simulink library "autodiff"  (R2017a)
settings: Solver=ode45  StartTime=0.0  StopTime=10.0  RelTol=1e-3  EnableMultiTasking=on
undefined symbols (not defined in the file or in its folder): trace
libraries: autodiff x19
settings Model: Creator=eruffaldi  LastModifiedBy=eruffaldi
settings DataIOCC: LimitDataPoints=on
settings OptimizationCC: LifeSpan=inf
settings DebuggingCC: AllowSymbolicDim=off  SFUnexpectedBacktrackingDiag=warning  SFNoUnconditionalDefaultTransitionDiag=warning  SFExecutionAtInitializationDiag=none
settings GRTTargetCC: TargetLangStandard=C89/C90 (ANSI)  GeneratePreprocessorConditionals=Disable all
settings ConfigComp: CovMetricSettings=dw  CovHtmlReporting=on  CovSaveCumulativeToWorkspaceVar=on  CovSaveSingleToWorkspaceVar=on  CovExternalEMLEnable=off

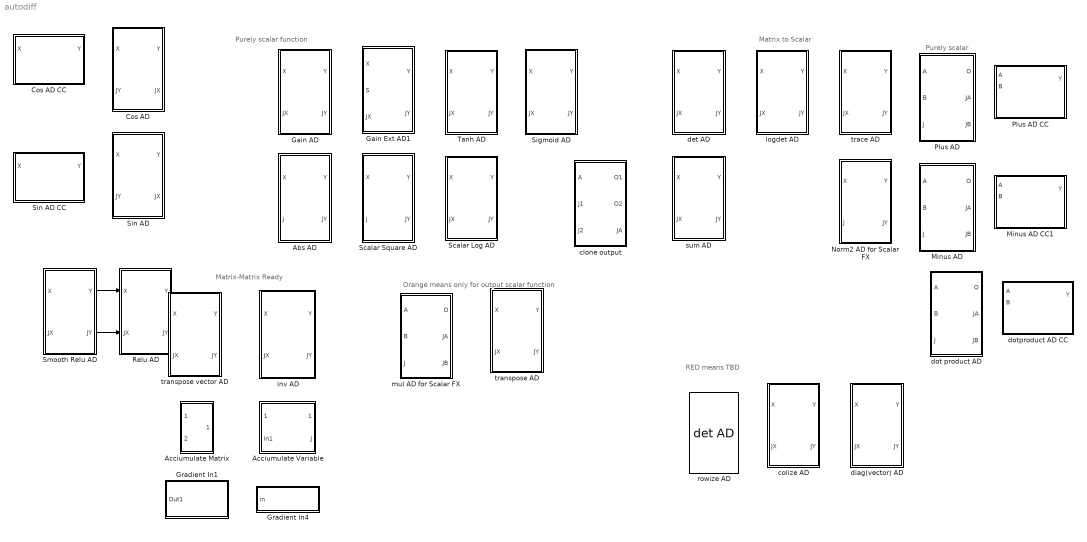
== system autodiff ==
  note: Matrix-Matrix Ready
  note: Purely scalar
  note: Matrix to Scalar
  note: Purely scalar function
  note: Orange means only for output scalar function
  note: RED means TBD
  Abs AD : Subsystem
  Acciumulate Matrix : Subsystem  mask{Inputs=2}
      mask Callback Inputs:
      | x = gcb;
      | s = gcb;
      | asked = max(1,str2num(get_param(gcb,'Inputs')));
      | 
      | bcon = [x '/Matrix Concatenate'];
      | actual = str2num(get_param(bcon,'NumInputs'));
      | 
      | if asked == actual
      | else
      | bconL = bcon(length(x)+2:end);
      | 
      | if asked > actual
      |     set_param(bcon,'NumInputs',num2str(asked));
      |     bin1 = ([x '/In1']);
      |     bsh1 = ([x '/Reshape1']);
      |     bin1L = bin1(length(x)+2:end);
      |     bsh1L = bsh1(length(x)+2:end);
      |     for I=actual+1:asked
      |         bin = sprintf([x '/In%d'],I);
      |         bsh = sprintf([x '/Reshape%d'],I);
      |         binL = bin(length(x)+2:end);
      |         bshL = bsh(length(x)+2:end);
      |         % clone In and Reshape
      |         add_block(bin1,bin);
      |         add_block(bsh1,bsh);
      |         add_line(s,[binL '/1'],[bshL '/1']);
      |         add_line(s,[bshL '/1'],[bconL sprintf('/%d',I)]);
      |     end
      | else
      |     % remove
      |     for I=actual:-1:asked+1
      |         bin = sprintf([x '/In%d'],I);
      |         bsh = sprintf([x '/Reshape%d'],I);
      |         binL = bin(length(x)+2:end);
      |         bshL = bsh(length(x)+2:end);
      | 
      |         try
      |         delete_line(s,[binL '/1'],[bshL '/1']);
      |         catch me
      |         end
      |         try
      |         delete_line(s,[bshL '/1'],[bconL sprintf('/%d',I)]);
      |         catch me
      |         end
      |         try
      |         delete_block(bin);
      |         catch me
      |         end
      |         try
      |         delete_block(bsh);
      |         catch me
      |         end
      |     end
      |     set_param(bcon,'NumInputs',num2str(asked));
      | end
      | end
  Acciumulate Variable : Subsystem  mask{Inputs=1}
      mask Callback Inputs:
      | x = gcb;
      | s = gcb;
      | asked = max(1,str2num(get_param(gcb,'Inputs')));
      | 
      | bcon = [x '/Matrix Concatenate'];
      | actual = str2num(get_param(bcon,'NumInputs'));
      | 
      | if asked == actual
      | else
      | bconL = bcon(length(x)+2:end);
      | 
      | if asked > actual
      |     set_param(bcon,'NumInputs',num2str(asked));
      |     bin1 = ([x '/In1']);
      |     bsh1 = ([x '/Reshape1']);
      |     bin1L = bin1(length(x)+2:end);
      |     bsh1L = bsh1(length(x)+2:end);
      |     for I=actual+1:asked
      |         bin = sprintf([x '/In%d'],I);
      |         bsh = sprintf([x '/Reshape%d'],I);
      |         binL = bin(length(x)+2:end);
      |         bshL = bsh(length(x)+2:end);
      |         % clone In and Reshape
      |         add_block(bin1,bin);
      |         add_block(bsh1,bsh);
      |         add_line(s,[binL '/1'],[bshL '/1']);
      |         add_line(s,[bshL '/1'],[bconL sprintf('/%d',I)]);
      |     end
      | else
      |     % remove
      |     for I=actual:-1:asked+1
      |         bin = sprintf([x '/In%d'],I);
      |         bsh = sprintf([x '/Reshape%d'],I);
      |         binL = bin(length(x)+2:end);
      |         bshL = bsh(length(x)+2:end);
      | 
      |         try
      |         delete_line(s,[binL '/1'],[bshL '/1']);
      |         catch me
      |         end
      |         try
      |         delete_line(s,[bshL '/1'],[bconL sprintf('/%d',I)]);
      |         catch me
      |         end
      |         try
      |         delete_block(bin);
      |         catch me
      |         end
      |         try
      |         delete_block(bsh);
      |         catch me
      |         end
      |     end
      |     set_param(bcon,'NumInputs',num2str(asked));
      | end
      | end
  Cos AD : Subsystem
  Cos AD CC : Subsystem
  Gain AD : Subsystem  mask{k=1}
      mask prompts: k "Gain Constant"
  Gain Ext AD1 : Subsystem
  Gradient In1 : Subsystem
  Gradient In4 : Subsystem
  Minus AD : Subsystem
  Minus AD CC1 : Subsystem
  Norm2 AD for Scalar FX : Subsystem
  "Plus AD " : Subsystem
  Plus AD CC : Subsystem
  Relu AD : Subsystem
  Scalar Log AD : Subsystem
  Scalar Square AD : Subsystem
  Sigmoid AD : Subsystem
  Sin AD : Subsystem
  Sin AD CC : Subsystem
  Smooth Relu AD : Subsystem
  Tanh AD : Subsystem
  clone output : Subsystem
  colize AD : Subsystem
  det AD : Subsystem
  diag(vector) AD : Subsystem
  dot product AD : Subsystem
  dotproduct AD CC : Subsystem
  inv AD : Subsystem
  logdet AD : Subsystem
  mul AD for Scalar FX : Subsystem
  rowize AD : autodiff/det AD
  sum AD : Subsystem
  trace AD : Subsystem
  transpose AD : Subsystem
  transpose vector AD : Subsystem
  wires:
  Smooth Relu AD/1(Y) -> Relu AD/1(X)
  Smooth Relu AD/2(JY) -> Relu AD/2(JX)

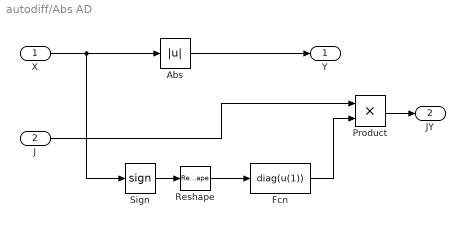
== system autodiff/Abs AD ==
  X : Inport
  J : Inport  Port=2
  Abs : Abs
  Fcn : Fcn  Expr=diag(u(1))
  Product : Product
  Reshape : Reshape  OutputDimensionality=Column vector (2-D)
  Sign : Signum
  Y : Outport
  JY : Outport  Port=2
  wires:
  Abs/1 -> Y/1
  X/1 -> Sign/1, Abs/1
  Sign/1 -> Reshape/1
  Product/1 -> JY/1
  Reshape/1 -> Fcn/1
  J/1 -> Product/1
  Fcn/1 -> Product/2

== system autodiff/Acciumulate Matrix ==
  In1 : Inport
  In2 : Inport  Port=2
  Matrix Concatenate : Concatenate  Mode=Multidimensional array  ConcatenateDimension=2
  Reshape1 : Reshape
  Reshape2 : Reshape
  ReshapeX : Reshape  OutputDimensionality=Derive from reference input port
  Sum of Elements : Sum  Inputs=+  CollapseMode=Specified dimension  CollapseDim=2
  Out1 : Outport
  wires:
  Sum of Elements/1 -> ReshapeX/1
  In1/1 -> ReshapeX/2, Reshape1/1
  Reshape1/1 -> Matrix Concatenate/1
  Matrix Concatenate/1 -> Sum of Elements/1
  ReshapeX/1 -> Out1/1
  In2/1 -> Reshape2/1
  Reshape2/1 -> Matrix Concatenate/2

== system autodiff/Acciumulate Variable ==
  note: InValue is the X that is passed by just due to visual style and it is size [m,n]
      |
      | The In# is automatically populated and it should be [p,q,m,n] that is [pq,mn] we
      | receive a set of k contributions [pq,mn] flatten as [pq mn, 1] then concatenate to [pq mn,k]
      | and sum obtaining as output [pq,mn] again
  InValue : Inport
  In1 : Inport  Port=2
  Matrix Concatenate : Concatenate  NumInputs=1  Mode=Multidimensional array  ConcatenateDimension=2
  Reshape1 : Reshape
  ReshapeX : Reshape  OutputDimensionality=Derive from reference input port
  Sum of Elements : Sum  Inputs=+  CollapseMode=Specified dimension  CollapseDim=2
  OutValue : Outport
  J : Outport  Port=2
  wires:
  Sum of Elements/1 -> ReshapeX/1
  In1/1 -> ReshapeX/2, Reshape1/1
  Reshape1/1 -> Matrix Concatenate/1
  Matrix Concatenate/1 -> Sum of Elements/1
  ReshapeX/1 -> J/1
  InValue/1 -> OutValue/1

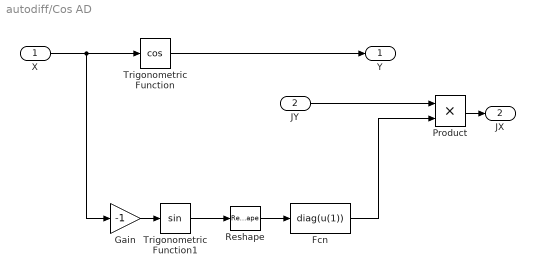
== system autodiff/Cos AD ==
  X : Inport
  JY : Inport  Port=2
  Fcn : Fcn  Expr=diag(u(1))
  Gain : Gain  Gain=-1
  Product : Product
  Reshape : Reshape  OutputDimensionality=Column vector (2-D)
  Trigonometric Function : Trigonometry  Operator=cos
  Trigonometric Function1 : Trigonometry
  Y : Outport
  JX : Outport  Port=2
  wires:
  Trigonometric Function/1 -> Y/1
  X/1 -> Gain/1, Trigonometric Function/1
  Product/1 -> JX/1
  Gain/1 -> Trigonometric Function1/1
  Trigonometric Function1/1 -> Reshape/1
  Fcn/1 -> Product/2
  JY/1 -> Product/1
  Reshape/1 -> Fcn/1

== system autodiff/Cos AD CC ==
  X : Inport
  Cos AD1 : autodiff/Cos AD
  Gradient In2 : autodiff/Gradient In4
  Gradient In3 : autodiff/Gradient In1
  JX : PMIOPort  Port=1  Side=Left
  JY : PMIOPort  Port=2  Side=Right
  Y : Outport
  wires:
  Gradient In3/1 -> Cos AD1/2
  Cos AD1/1 -> Y/1
  X/1 -> Cos AD1/1
  Cos AD1/2 -> Gradient In2/1
  connections:
  Gradient In2/RConn1 -- JX/RConn1
  Gradient In3/LConn1 -- JY/RConn1

== system autodiff/Gain AD ==
  X : Inport
  JX : Inport  Port=2
  Gain1 : Gain  Gain=k
  Gain2 : Gain  Gain=k
  Y : Outport
  JY : Outport  Port=2
  wires:
  Gain1/1 -> Y/1
  X/1 -> Gain1/1
  Gain2/1 -> JY/1
  JX/1 -> Gain2/1

== system autodiff/Gain Ext AD1 ==
  X : Inport
  S : Inport  Port=2
  JX : Inport  Port=3
  Product : Product
  Product1 : Product
  Signal Specification : SignalSpecification  Dimensions=1
  Y : Outport
  JY : Outport  Port=2
  wires:
  Product1/1 -> Y/1
  X/1 -> Product1/1
  Product/1 -> JY/1
  JX/1 -> Product/2
  S/1 -> Signal Specification/1
  Signal Specification/1 -> Product1/2, Product/1

== system autodiff/Gradient In1 ==
  Ground : Ground
  Two-Way Connection : TwoWayConnection
  J out : PMIOPort  Port=1  Side=Left
  Out1 : Outport
  wires:
  Two-Way Connection/1 -> Out1/1
  Ground/1 -> Two-Way Connection/1
  connections:
  J out/RConn1 -- Two-Way Connection/RConn1

== system autodiff/Gradient In4 ==
  " in" : Inport
  Terminator : Terminator
  Two-Way Connection : TwoWayConnection
  J out : PMIOPort  Port=1  Side=Right
  wires:
  " in"/1 -> Two-Way Connection/1
  Two-Way Connection/1 -> Terminator/1
  connections:
  J out/RConn1 -- Two-Way Connection/RConn1

== system autodiff/Minus AD ==
  A : Inport
  B : Inport  Port=2
  J : Inport  Port=3
  Add : Sum  Inputs=+-
  Gain : Gain  Gain=-1
  O : Outport
  JA : Outport  Port=2
  JB : Outport  Port=3
  wires:
  Add/1 -> O/1
  A/1 -> Add/1
  B/1 -> Add/2
  J/1 -> Gain/1, JA/1
  Gain/1 -> JB/1

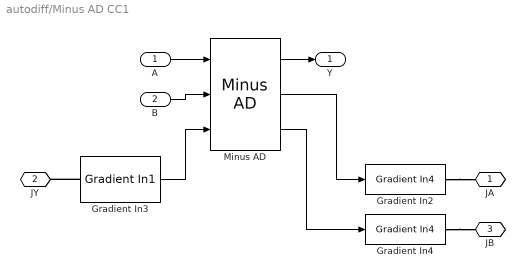
== system autodiff/Minus AD CC1 ==
  A : Inport
  B : Inport  Port=2
  Gradient In2 : autodiff/Gradient In4
  Gradient In3 : autodiff/Gradient In1
  Gradient In4 : autodiff/Gradient In4
  Minus AD : autodiff/Minus AD
  JA : PMIOPort  Port=1  Side=Left
  JY : PMIOPort  Port=2  Side=Right
  JB : PMIOPort  Port=3  Side=Left
  Y : Outport
  wires:
  Gradient In3/1 -> Minus AD/3
  Minus AD/1 -> Y/1
  A/1 -> Minus AD/1
  B/1 -> Minus AD/2
  Minus AD/2 -> Gradient In2/1
  Minus AD/3 -> Gradient In4/1
  connections:
  Gradient In2/RConn1 -- JA/RConn1
  Gradient In3/LConn1 -- JY/RConn1
  Gradient In4/RConn1 -- JB/RConn1

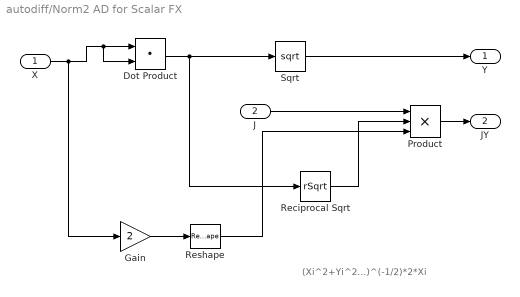
== system autodiff/Norm2 AD for Scalar FX ==
  note: (Xi^2+Yi^2...)^(-1/2)*2*Xi
  X : Inport
  J : Inport  Port=2
  Dot Product : DotProduct  InputSameDT=on  OutDataTypeStr=Inherit: Inherit via internal rule
  Gain : Gain  Gain=2
  Product : Product  Inputs=3
  Reciprocal Sqrt : Sqrt  Operator=rSqrt  SaturateOnIntegerOverflow=on
  Reshape : Reshape  OutputDimensionality=Row vector (2-D)
  Sqrt : Sqrt  SaturateOnIntegerOverflow=on
  Y : Outport
  JY : Outport  Port=2
  wires:
  X/1 -> Gain/1, Dot Product/2, Dot Product/1
  Product/1 -> JY/1
  Dot Product/1 -> Reciprocal Sqrt/1, Sqrt/1
  Sqrt/1 -> Y/1
  J/1 -> Product/1
  Reciprocal Sqrt/1 -> Product/2
  Gain/1 -> Reshape/1
  Reshape/1 -> Product/3

== system autodiff/Plus AD  ==
  A : Inport
  B : Inport  Port=2
  J : Inport  Port=3
  Add : Sum
  O : Outport
  JA : Outport  Port=2
  JB : Outport  Port=3
  wires:
  Add/1 -> O/1
  A/1 -> Add/1
  B/1 -> Add/2
  J/1 -> JB/1, JA/1

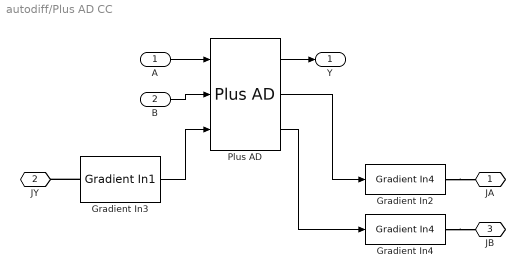
== system autodiff/Plus AD CC ==
  A : Inport
  B : Inport  Port=2
  Gradient In2 : autodiff/Gradient In4
  Gradient In3 : autodiff/Gradient In1
  Gradient In4 : autodiff/Gradient In4
  "Plus AD " : autodiff/Plus AD  
  JA : PMIOPort  Port=1  Side=Left
  JY : PMIOPort  Port=2  Side=Right
  JB : PMIOPort  Port=3  Side=Left
  Y : Outport
  wires:
  Gradient In3/1 -> "Plus AD "/3
  "Plus AD "/1 -> Y/1
  A/1 -> "Plus AD "/1
  B/1 -> "Plus AD "/2
  "Plus AD "/2 -> Gradient In2/1
  "Plus AD "/3 -> Gradient In4/1
  connections:
  Gradient In2/RConn1 -- JA/RConn1
  Gradient In3/LConn1 -- JY/RConn1
  Gradient In4/RConn1 -- JB/RConn1

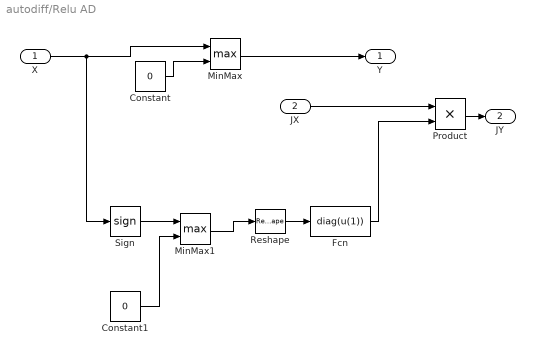
== system autodiff/Relu AD ==
  X : Inport
  JX : Inport  Port=2
  Constant : Constant  Value=0
  Constant1 : Constant  Value=0
  Fcn : Fcn  Expr=diag(u(1))
  MinMax : MinMax  Function=max  Inputs=2
  MinMax1 : MinMax  Function=max  Inputs=2
  Product : Product
  Reshape : Reshape  OutputDimensionality=Column vector (2-D)
  Sign : Signum
  Y : Outport
  JY : Outport  Port=2
  wires:
  MinMax/1 -> Y/1
  X/1 -> Sign/1, MinMax/1
  Product/1 -> JY/1
  MinMax1/1 -> Reshape/1
  Fcn/1 -> Product/2
  JX/1 -> Product/1
  Reshape/1 -> Fcn/1
  Constant/1 -> MinMax/2
  Sign/1 -> MinMax1/1
  Constant1/1 -> MinMax1/2

== system autodiff/Scalar Log AD ==
  X : Inport
  JX : Inport  Port=2
  Fcn : Fcn  Expr=diag(u(1))
  Fcn1 : Fcn  Expr=1./u(1)
  Math Function : Math  Operator=log  SaturateOnIntegerOverflow=on
  Product : Product
  Reshape : Reshape  OutputDimensionality=Column vector (2-D)
  Y : Outport
  JY : Outport  Port=2
  wires:
  Math Function/1 -> Y/1
  X/1 -> Fcn1/1, Math Function/1
  Product/1 -> JY/1
  Fcn1/1 -> Reshape/1
  Fcn/1 -> Product/2
  JX/1 -> Product/1
  Reshape/1 -> Fcn/1

== system autodiff/Scalar Square AD ==
  X : Inport
  J : Inport  Port=2
  Fcn : Fcn  Expr=diag(u(1))
  Fcn1 : Fcn  Expr=u(1).^2
  Gain : Gain  Gain=2
  Product : Product
  Reshape : Reshape  OutputDimensionality=Column vector (2-D)
  Y : Outport
  JY : Outport  Port=2
  wires:
  Fcn1/1 -> Y/1
  X/1 -> Gain/1, Fcn1/1
  Gain/1 -> Reshape/1
  Product/1 -> JY/1
  Reshape/1 -> Fcn/1
  J/1 -> Product/1
  Fcn/1 -> Product/2

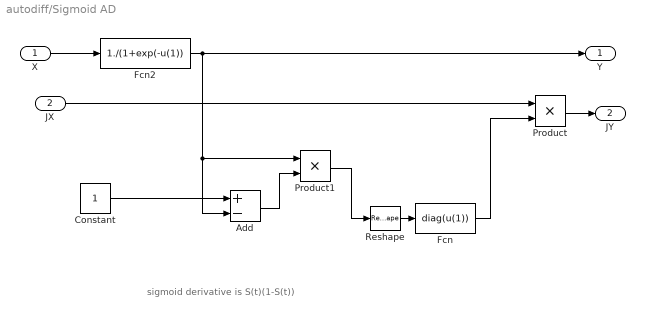
== system autodiff/Sigmoid AD ==
  note: sigmoid derivative is S(t)(1-S(t))
  X : Inport
  JX : Inport  Port=2
  Add : Sum  Inputs=+-
  Constant : Constant
  Fcn : Fcn  Expr=diag(u(1))
  Fcn2 : Fcn  Expr=1./(1+exp(-u(1))
  Product : Product
  Product1 : Product
  Reshape : Reshape  OutputDimensionality=Column vector (2-D)
  Y : Outport
  JY : Outport  Port=2
  wires:
  Product/1 -> JY/1
  Fcn/1 -> Product/2
  JX/1 -> Product/1
  Reshape/1 -> Fcn/1
  X/1 -> Fcn2/1
  Fcn2/1 -> Add/2, Product1/1, Y/1
  Constant/1 -> Add/1
  Add/1 -> Product1/2
  Product1/1 -> Reshape/1

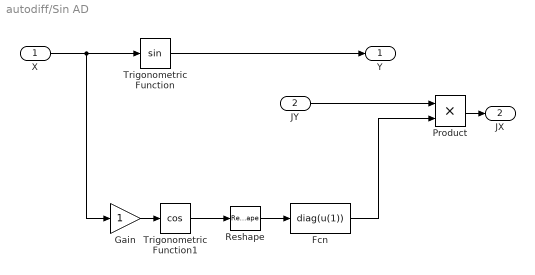
== system autodiff/Sin AD ==
  X : Inport
  JY : Inport  Port=2
  Fcn : Fcn  Expr=diag(u(1))
  Gain : Gain
  Product : Product
  Reshape : Reshape  OutputDimensionality=Column vector (2-D)
  Trigonometric Function : Trigonometry
  Trigonometric Function1 : Trigonometry  Operator=cos
  Y : Outport
  JX : Outport  Port=2
  wires:
  Trigonometric Function/1 -> Y/1
  X/1 -> Gain/1, Trigonometric Function/1
  Product/1 -> JX/1
  Gain/1 -> Trigonometric Function1/1
  Trigonometric Function1/1 -> Reshape/1
  Fcn/1 -> Product/2
  JY/1 -> Product/1
  Reshape/1 -> Fcn/1

== system autodiff/Sin AD CC ==
  X : Inport
  Gradient In2 : autodiff/Gradient In4
  Gradient In3 : autodiff/Gradient In1
  Sin AD : autodiff/Sin AD
  JX : PMIOPort  Port=1  Side=Left
  JY : PMIOPort  Port=2  Side=Right
  Y : Outport
  wires:
  Gradient In3/1 -> Sin AD/2
  Sin AD/1 -> Y/1
  X/1 -> Sin AD/1
  Sin AD/2 -> Gradient In2/1
  connections:
  Gradient In2/RConn1 -- JX/RConn1
  Gradient In3/LConn1 -- JY/RConn1

== system autodiff/Smooth Relu AD ==
  X : Inport
  JX : Inport  Port=2
  Fcn : Fcn  Expr=diag(u(1))
  Fcn1 : Fcn  Expr=log(1+exp(u(1))
  Fcn2 : Fcn  Expr=1./(1+exp(-u(1))
  Product : Product
  Reshape : Reshape  OutputDimensionality=Column vector (2-D)
  Y : Outport
  JY : Outport  Port=2
  wires:
  Fcn1/1 -> Y/1
  X/1 -> Fcn2/1, Fcn1/1
  Product/1 -> JY/1
  Fcn2/1 -> Reshape/1
  Fcn/1 -> Product/2
  JX/1 -> Product/1
  Reshape/1 -> Fcn/1

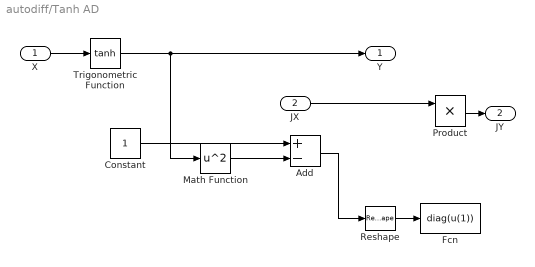
== system autodiff/Tanh AD ==
  X : Inport
  JX : Inport  Port=2
  Add : Sum  Inputs=+-
  Constant : Constant
  Fcn : Fcn  Expr=diag(u(1))
  Math Function : Math  Operator=square  SaturateOnIntegerOverflow=on
  Product : Product
  Reshape : Reshape  OutputDimensionality=Column vector (2-D)
  Trigonometric Function : Trigonometry  Operator=tanh
  Y : Outport
  JY : Outport  Port=2
  wires:
  Trigonometric Function/1 -> Math Function/1, Y/1
  X/1 -> Trigonometric Function/1
  Product/1 -> JY/1
  JX/1 -> Product/1
  Reshape/1 -> Fcn/1
  Constant/1 -> Add/1
  Add/1 -> Reshape/1
  Math Function/1 -> Add/2

== system autodiff/clone output ==
  note: J is [p,q,1,1]=[pq,1]
      | outputs JA and JB are [pq,m]
  A : Inport
  J1 : Inport  Port=2
  "J2 " : Inport  Port=3
  Add : Sum
  O1 : Outport
  O2 : Outport  Port=2
  JA : Outport  Port=3
  wires:
  J1/1 -> Add/1
  Add/1 -> JA/1
  A/1 -> O2/1, O1/1
  "J2 "/1 -> Add/2

== system autodiff/colize AD ==
  X : Inport
  JX : Inport  Port=2
  Fcn : Fcn  Expr=det(u(1))
  Fcn1 : Fcn  Expr=inv(u(1))
  Product : Product  Inputs=3
  Reshape : Reshape  OutputDimensionality=Row vector (2-D)
  Y : Outport
  JY : Outport  Port=2
  wires:
  Fcn/1 -> Product/1, Y/1
  Product/1 -> JY/1
  X/1 -> Fcn1/1, Fcn/1
  Fcn1/1 -> Reshape/1
  JX/1 -> Product/2
  Reshape/1 -> Product/3

== system autodiff/det AD ==
  X : Inport
  JX : Inport  Port=2
  Fcn : Fcn  Expr=det(u(1))
  Fcn1 : Fcn  Expr=inv(u(1))
  Product : Product  Inputs=3
  Reshape : Reshape  OutputDimensionality=Row vector (2-D)
  Y : Outport
  JY : Outport  Port=2
  wires:
  Fcn/1 -> Product/1, Y/1
  Product/1 -> JY/1
  X/1 -> Fcn1/1, Fcn/1
  Fcn1/1 -> Reshape/1
  JX/1 -> Product/2
  Reshape/1 -> Product/3

== system autodiff/diag(vector) AD ==
  note: Takes a vector and builds a diagonal matrix
      |
      | Incoming JX is [pq,nn] and JY is [pq,n 1] so we need [nn,n]]
  X : Inport
  JX : Inport  Port=2
  Fcn : Fcn  Expr=diag(u(1))
  Product : Product
  Reshape : Reshape  OutputDimensionality=Row vector (2-D)
  Y : Outport
  JY : Outport  Port=2
  wires:
  Fcn/1 -> Y/1
  Product/1 -> JY/1
  X/1 -> Fcn/1
  ? -> Reshape/1
  JX/1 -> Product/1

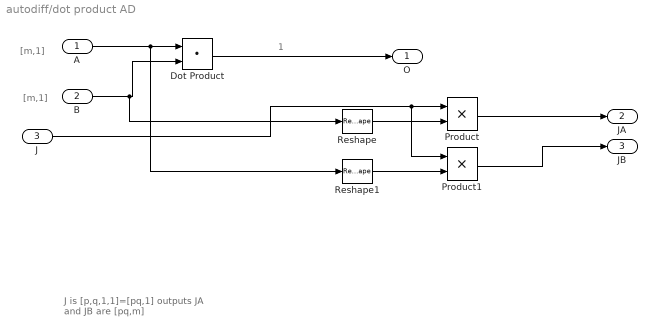
== system autodiff/dot product AD ==
  note: 1
  note: [m,1]
  note: [m,1]
  note: J is [p,q,1,1]=[pq,1]
      | outputs JA and JB are [pq,m]
  A : Inport
  B : Inport  Port=2
  J : Inport  Port=3
  Dot Product : DotProduct  InputSameDT=on  OutDataTypeStr=Inherit: Inherit via internal rule
  Product : Product
  Product1 : Product
  Reshape : Reshape  OutputDimensionality=Row vector (2-D)
  Reshape1 : Reshape  OutputDimensionality=Row vector (2-D)
  O : Outport
  JA : Outport  Port=2
  JB : Outport  Port=3
  wires:
  Dot Product/1 -> O/1
  A/1 -> Reshape1/1, Dot Product/1
  B/1 -> Reshape/1, Dot Product/2
  J/1 -> Product1/1, Product/1
  Product/1 -> JA/1
  Product1/1 -> JB/1
  Reshape/1 -> Product/2
  Reshape1/1 -> Product1/2

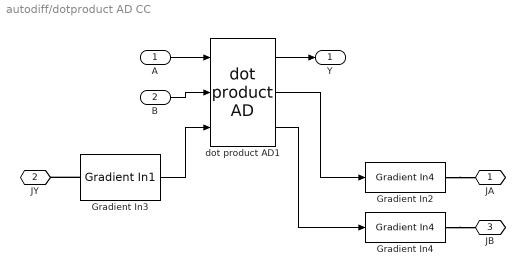
== system autodiff/dotproduct AD CC ==
  A : Inport
  B : Inport  Port=2
  Gradient In2 : autodiff/Gradient In4
  Gradient In3 : autodiff/Gradient In1
  Gradient In4 : autodiff/Gradient In4
  dot product AD1 : autodiff/dot product AD
  JA : PMIOPort  Port=1  Side=Left
  JY : PMIOPort  Port=2  Side=Right
  JB : PMIOPort  Port=3  Side=Left
  Y : Outport
  wires:
  Gradient In3/1 -> dot product AD1/3
  dot product AD1/1 -> Y/1
  A/1 -> dot product AD1/1
  B/1 -> dot product AD1/2
  dot product AD1/2 -> Gradient In2/1
  dot product AD1/3 -> Gradient In4/1
  connections:
  Gradient In2/RConn1 -- JA/RConn1
  Gradient In3/LConn1 -- JY/RConn1
  Gradient In4/RConn1 -- JB/RConn1

== system autodiff/inv AD ==
  note: Jx = Jy*(-kron(y',y));
  X : Inport
  JX : Inport  Port=2
  Fcn : Fcn  Expr=inv(u(1))
  Fcn1 : Fcn  Expr=-kron(u(1)',u(1))
  Product : Product
  Y : Outport
  JY : Outport  Port=2
  wires:
  Fcn/1 -> Fcn1/1, Y/1
  Product/1 -> JY/1
  X/1 -> Fcn/1
  Fcn1/1 -> Product/2
  JX/1 -> Product/1

== system autodiff/logdet AD ==
  X : Inport
  JX : Inport  Port=2
  Fcn : Fcn  Expr=det(u(1))
  Fcn1 : Fcn  Expr=inv(u(1))
  Product : Product
  Reshape : Reshape  OutputDimensionality=Row vector (2-D)
  Y : Outport
  JY : Outport  Port=2
  wires:
  Fcn/1 -> Y/1
  Product/1 -> JY/1
  X/1 -> Fcn1/1, Fcn/1
  Fcn1/1 -> Reshape/1
  JX/1 -> Product/1
  Reshape/1 -> Product/2

== system autodiff/mul AD for Scalar FX ==
  note: [q,n]
  note: [m,q]
  note: [m,n]
  note: [q,n]
  note: [m,q]
  note: Coming from parent it is sized [m,n]
  A : Inport
  B : Inport  Port=2
  J : Inport  Port=3
  Divide : Product  Inputs=**  Multiplication=Matrix(*)
  MATLAB Function : MATLAB Function  TreatAsAtomicUnit=on
  MATLAB Function1 : MATLAB Function  TreatAsAtomicUnit=on
  O : Outport
  JA : Outport  Port=2
  JB : Outport  Port=3
  wires:
  Divide/1 -> O/1
  A/1 -> MATLAB Function1/1(X), MATLAB Function/1(X), Divide/1
  MATLAB Function1/1(y) -> JB/1
  MATLAB Function/1(y) -> JA/1
  B/1 -> MATLAB Function1/2(Y), MATLAB Function/2(Y), Divide/2
  J/1 -> MATLAB Function1/3(J), MATLAB Function/3(J)

== system autodiff/sum AD ==
  note: X is [m.n] output is 1
      | JX is [p,q,1,1] output is [p,q,m,n] that is [pq,mn]
      | so we multiply [pq,1] [1,mn]
  X : Inport
  JX : Inport  Port=2
  Fcn1 : Fcn  Expr=ones(1,length(u(1)))
  Product : Product
  Sum of Elements : Sum  Inputs=+
  Y : Outport
  JY : Outport  Port=2
  wires:
  Sum of Elements/1 -> Y/1
  Product/1 -> JY/1
  X/1 -> Sum of Elements/1, Fcn1/1
  JX/1 -> Product/1
  Fcn1/1 -> Product/2

== system autodiff/trace AD ==
  X : Inport
  JX : Inport  Port=2
  Fcn : Fcn  Expr=trace(u(1))
  Fcn1 : Fcn  Expr=eye(length(u(1)))
  Product : Product
  Reshape : Reshape  OutputDimensionality=Row vector (2-D)
  Y : Outport
  JY : Outport  Port=2
  wires:
  Fcn/1 -> Y/1
  Product/1 -> JY/1
  X/1 -> Fcn1/1, Fcn/1
  Fcn1/1 -> Reshape/1
  JX/1 -> Product/1
  Reshape/1 -> Product/2

== system autodiff/transpose AD ==
  note: We would suffice with a constant block that can be modified at InitFcn
  note: function Tmn = dtranspose(V)
      |             n = size(V,1);
      |             m = size(V,2);
      |             d = m*n;
      |             Tmn = zeros(d,d);
      |
      |             i = 1:d;
      |             rI = 1+m.*(i-1)-(m*n-1).*floor((i-1)./n);
      |             I1s = sub2ind([d d],rI,1:d);
      |             Tmn(I1s) = 1;
      |             Tmn = Tmn';
      |         end
  X : Inport
  JX : Inport  Port=2
  Level-2 MATLAB S-Function : M-S-Function  FunctionName=dtranspose_sfun
  Permute Dimensions : PermuteDimensions
  Product : Product
  Y : Outport
  JY : Outport  Port=2
  wires:
  Permute Dimensions/1 -> Y/1
  X/1 -> Level-2 MATLAB S-Function/1, Permute Dimensions/1
  Product/1 -> JY/1
  Level-2 MATLAB S-Function/1 -> Product/2
  JX/1 -> Product/1

== system autodiff/transpose vector AD ==
  note: The incoming JX is [p,q, m, 1] and the output [p,q,1,m]
      | The compact form becomes [pq,m] as [pq,m] so no changes
  X : Inport
  JX : Inport  Port=2
  Permute Dimensions : PermuteDimensions
  Y : Outport
  JY : Outport  Port=2
  wires:
  Permute Dimensions/1 -> Y/1
  X/1 -> Permute Dimensions/1
  JX/1 -> JY/1

== matlab function autodiff/mul AD for Scalar FX/MATLAB Function1 ==
  data: X input; y output; Y input; J input
function y = fcn(X,Y,J)
%#codegen

y = repmat(reshape(sum(X,1),size(X,2),1),1,size(Y,2));
if length(J) == 1
    y = J*y;
else
    y = repmat(sum(J,1),size(Y,1),1).*y;
end

== matlab function autodiff/mul AD for Scalar FX/MATLAB Function ==
  data: X input; y output; Y input; J input
function y = fcn(X,Y,J)
%#codegen

y = repmat(reshape(sum(Y,2),1,size(Y,1)),size(X,1),1);
if length(J) == 1
    y = J*y;
else
    y = repmat(sum(J,2),1,size(X,2)).*y;
end
